simulink model "untitled"  (R2017b)
settings: Solver=VariableStepAuto  StartTime=0.0  StopTime=10.0  RelTol=1e-3
undefined symbols (not defined in the file or in its folder): g, J, m, R
settings Model: Creator=ge_mathi  LastModifiedBy=ge_mathi

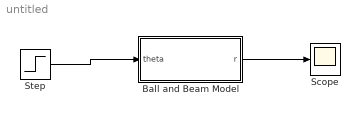
== system untitled ==
  Ball and Beam Model : Subsystem
  Scope : Scope
  Step : Step  SampleTime=0
  wires:
  Step/1 -> Ball and Beam Model/1(theta)
  Ball and Beam Model/1("r ") -> Scope/1

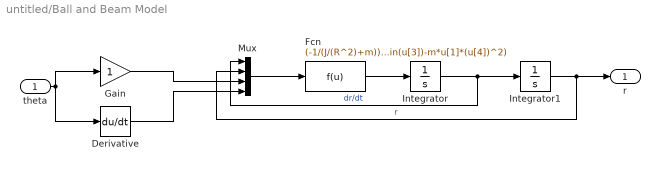
== system untitled/Ball and Beam Model ==
  theta : Inport
  Derivative : Derivative
  Fcn : Fcn  Expr=(-1/(J/(R^2)+m))*(m*g*sin(u[3])-m*u[1]*(u[4])^2)
  Gain : Gain
  Integrator : Integrator
  Integrator1 : Integrator
  Mux : Mux
  "r " : Outport
  wires:
  Integrator1/1 -> Mux/2, "r "/1  "r"
  Integrator/1 -> Mux/1, Integrator1/1  "dr/dt"
  Mux/1 -> Fcn/1
  theta/1 -> Derivative/1, Gain/1
  Gain/1 -> Mux/3
  Derivative/1 -> Mux/4
  Fcn/1 -> Integrator/1
